simulink model "porte_avion_obs"  (R2025b)
settings: Solver=VariableStepAuto  StartTime=0.0  StopTime=500  RelTol=1e-3
values from neighbouring files (symbols this model uses):
  A = [0 1 0 0 ... (first row only)    [porte_avion.m]
  A_obs = [A           E ... (first row only)    [porte_avion.m]
  B = [0 ... (first row only)    [porte_avion.m]
  B_obs = [B; 0]    [porte_avion.m]
  C = [0 0 1 0]    [porte_avion.m]
  C2 = [1 0 0 0 ... (first row only)    [porte_avion.m]
  C_obs = [C2 zeros(2, 1)]    [porte_avion.m]
  D = 0    [porte_avion.m]
  D2 = [0 ... (first row only)    [porte_avion.m]
  H = -pinv((C) * ((A - B*K) \ B))    [porte_avion.m]
  K = place(A, B, poles_cmd)    [porte_avion.m]
  Ki = -2000    [porte_avion.m]
  L = place(A', C', poles_obs)'    [porte_avion.m]
  L_obs = place(A_obs', C_obs', [-2, -2.5, -3, -3.5, -4])'    [porte_avion.m]
  omega_pert = 0.1    [porte_avion.m]
  r = 0    [porte_avion.m]
  X_0 = [x_0 ... (first row only)    [porte_avion.m]
settings Model: Creator=vikfo  LastModifiedBy=victor

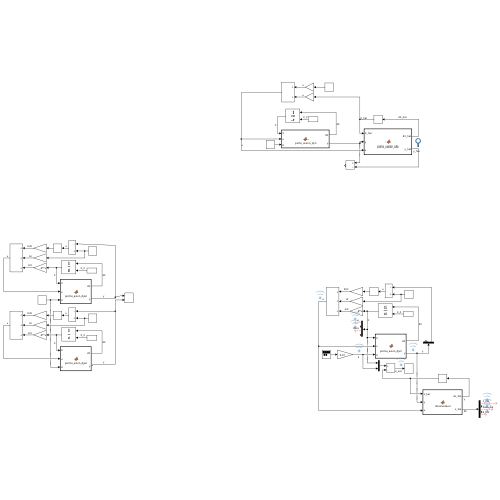
[thumbnail: Simulink's stored preview of the top-level diagram]
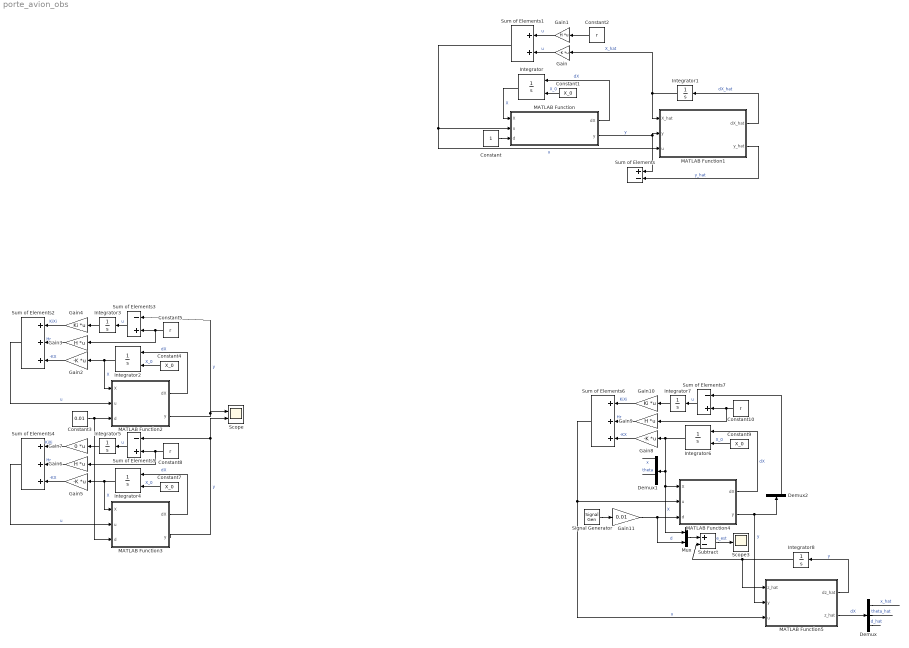
== system porte_avion_obs ==
  Constant : Constant
  Constant{1,4,7,9} (4 alike) : Constant  Value=X_0
  Constant{2,5,8,10} (4 alike) : Constant  Value=r
  Constant3 : Constant  Value=0.01
  Demux : Demux  Outputs=5
  Demux1 : Demux
  Demux2 : Demux  Outputs=2
  Gain{,2,5,8} (4 alike) : Gain  Gain=-K  Multiplication=Matrix(K*u)
  Gain{1,3,6,9} (4 alike) : Gain  Gain=H  Multiplication=Matrix(K*u)
  Gain10 : Gain  Gain=Ki  Multiplication=Matrix(K*u)
  Gain11 : Gain  Gain=0.01
  Gain4 : Gain  Gain=Ki  Multiplication=Matrix(K*u)
  Gain7 : Gain  Gain=0  Multiplication=Matrix(K*u)
  Integrator{,2,4,6} (4 alike) : Integrator  InitialConditionSource=external
  Integrator{1,3,5,7} (4 alike) : Integrator
  Integrator8 : Integrator  InitialCondition=zeros(5, 1)
  MATLAB Function : MATLAB Function  TreatAsAtomicUnit=on
  MATLAB Function1 : MATLAB Function  TreatAsAtomicUnit=on
  MATLAB Function2 : MATLAB Function  TreatAsAtomicUnit=on
  MATLAB Function3 : MATLAB Function  TreatAsAtomicUnit=on
  MATLAB Function4 : MATLAB Function  TreatAsAtomicUnit=on
  MATLAB Function5 : MATLAB Function  TreatAsAtomicUnit=on
  Mux : Mux  Inputs=[4 1]
  Scope : Scope  NumInputPorts=2
      settings: ActiveDisplayYMinimum=-1.369875447599938  ActiveDisplayYMaximum=0.62027967456851218
  Scope3 : Scope
      settings: ActiveDisplayYMinimum=-1.369875447599938  ActiveDisplayYMaximum=0.62027967456851218  DataLoggingVariableName=ScopeData3
  Signal Generator : SignalGenerator  Frequency=omega_pert  Units=rad/sec
  Subtract : Sum  Inputs=+-
  Sum of Elements : Sum  Inputs=+-
  Sum of Elements1 : Sum
  Sum of Elements2 : Sum  Inputs=+++
  Sum of Elements3 : Sum  Inputs=-+
  Sum of Elements4 : Sum  Inputs=+++
  Sum of Elements5 : Sum  Inputs=-+
  Sum of Elements6 : Sum  Inputs=+++
  Sum of Elements7 : Sum  Inputs=-+
  wires:
  MATLAB Function/1(dX) -> Integrator/1  "dX"
  Integrator/1 -> MATLAB Function/1(X)  "X"
  Sum of Elements1/1 -> MATLAB Function1/3(u), MATLAB Function/2(u)  "u"
  MATLAB Function/2(y) -> MATLAB Function1/2(y), Sum of Elements/1  "y"
  MATLAB Function1/1(dX_hat) -> Integrator1/1  "dX_hat"
  Integrator1/1 -> Gain/1, MATLAB Function1/1(X_hat)  "X_hat"
  Constant1/1 -> Integrator/2  "X_0"
  MATLAB Function1/2(y_hat) -> Sum of Elements/2  "y_hat"
  Constant/1 -> MATLAB Function/3(d)
  Constant2/1 -> Gain1/1
  Gain1/1 -> Sum of Elements1/1  "u"
  Gain/1 -> Sum of Elements1/2  "u"
  Constant5/1 -> Gain3/1, Sum of Elements3/2
  Gain3/1 -> Sum of Elements2/2  "Hr"
  Integrator2/1 -> MATLAB Function2/1(X), Gain2/1  "X"
  MATLAB Function2/2(y) -> Sum of Elements3/1, Scope/1  "y"
  Gain2/1 -> Sum of Elements2/3  "-KX"
  Constant4/1 -> Integrator2/2  "X_0"
  MATLAB Function2/1(dX) -> Integrator2/1  "dX"
  Sum of Elements2/1 -> MATLAB Function2/2(u)  "u"
  Gain4/1 -> Sum of Elements2/1  "KiXi"
  Integrator3/1 -> Gain4/1
  Sum of Elements3/1 -> Integrator3/1  "u"
  Gain5/1 -> Sum of Elements4/3  "-KX"
  Sum of Elements4/1 -> MATLAB Function3/2(u)  "u"
  Constant3/1 -> MATLAB Function3/3(d), MATLAB Function2/3(d)
  MATLAB Function3/1(dX) -> Integrator4/1  "dX"
  Gain7/1 -> Sum of Elements4/1  "KiXi"
  MATLAB Function3/2(y) -> Scope/2, Sum of Elements5/1  "y"
  Constant7/1 -> Integrator4/2  "X_0"
  Sum of Elements5/1 -> Integrator5/1  "u"
  Gain6/1 -> Sum of Elements4/2  "Hr"
  Integrator5/1 -> Gain7/1
  Integrator4/1 -> MATLAB Function3/1(X), Gain5/1  "X"
  Constant8/1 -> Gain6/1, Sum of Elements5/2
  Gain8/1 -> Sum of Elements6/3  "-KX"
  Sum of Elements6/1 -> MATLAB Function4/2(u), MATLAB Function5/3(u)  "u"
  MATLAB Function4/1(dX) -> Integrator6/1  "dX"
  Gain10/1 -> Sum of Elements6/1  "KiXi"
  MATLAB Function4/2(y) -> Demux2/1, MATLAB Function5/2(y)  "y"
  Constant9/1 -> Integrator6/2  "X_0"
  Sum of Elements7/1 -> Integrator7/1  "u"
  Gain9/1 -> Sum of Elements6/2  "Hr"
  Integrator7/1 -> Gain10/1
  Integrator6/1 -> Mux/1, MATLAB Function4/1(X), Demux1/1, Gain8/1  "X"
  Constant10/1 -> Gain9/1, Sum of Elements7/2
  Gain11/1 -> Mux/2, MATLAB Function4/3(d)  "d"
  MATLAB Function5/1(dz_hat) -> Integrator8/1  "y"
  Integrator8/1 -> MATLAB Function5/1("z_hat "), Subtract/2
  MATLAB Function5/2(z_hat) -> Demux/1  "dX"
  Demux/5 -> ?  "d_hat"
  Demux/1 -> ?  "x_hat"
  Demux/3 -> ?  "theta_hat"
  Demux1/1 -> ?  "x"
  Demux1/3 -> ?  "theta"
  Demux2/2 -> Sum of Elements7/1
  Mux/1 -> Subtract/1
  Subtract/1 -> Scope3/1  "e_est"
  Signal Generator/1 -> Gain11/1

== matlab function porte_avion_obs/MATLAB Function1 ==
  data: X_hat input; y input; u input; dX_hat output; A parameter; B parameter; C parameter; D parameter; y_hat output; L parameter
function [dX_hat, y_hat]  = porte_avion_obs(X_hat, y, u, A, B, C, D, L)

y_hat = C*X_hat + D*u;

dX_hat = zeros(4, 1);

dX_hat = A*X_hat + B*u + L*(y-y_hat);
end

== matlab function porte_avion_obs/MATLAB Function ==
  data: X input; u input; d input; dX output; y output; A parameter; B parameter; C parameter; D parameter; E parameter
function [dX, y]= porte_avion_dyn(X, u, d, A, B, C, D, E)
dX = A*X + B*u + E*d;
y = C*X + D*u;
end

== matlab function porte_avion_obs/MATLAB Function2 ==
  data: X input; u input; d input; dX output; y output; A parameter; B parameter; C parameter; D parameter; E parameter
function [dX, y]= porte_avion_dyn(X, u, d, A, B, C, D, E)
dX = A*X + B*u + E*d;
y = C*X + D*u;
end

== matlab function porte_avion_obs/MATLAB Function3 ==
  data: X input; u input; d input; dX output; y output; A parameter; B parameter; C parameter; D parameter; E parameter
function [dX, y]= porte_avion_dyn(X, u, d, A, B, C, D, E)
dX = A*X + B*u + E*d;
y = C*X + D*u;
end

== matlab function porte_avion_obs/MATLAB Function4 ==
  data: X input; u input; d input; dX output; y output; A parameter; B parameter; C2 parameter; D2 parameter; E parameter
function [dX, y]= porte_avion_dyn(X, u, d, A, B, C2, D2, E)
dX = A*X + B*u + E*d;
y = C2*X + D2*u;
end

== matlab function porte_avion_obs/MATLAB Function5 ==
  data: dz_hat output; z_hat input; y input; u input; A_obs parameter; z_hat output; B_obs parameter; C_obs parameter; L_obs parameter
function [dz_hat, z_hat]= observateur(z_hat, y, u, A_obs, B_obs, C_obs, L_obs)
dz_hat = zeros(5, 1);
dz_hat = A_obs*z_hat + B_obs*u + L_obs*(y - C_obs*z_hat);
end
